simulink model "eml_2nd_order_filter_vectorized"  (Simulink 7.3)
settings: Solver=FixedStepDiscrete  StartTime=0.0  StopTime=0  RelTol=1e-3
values from neighbouring files (symbols this model uses):
  den = [1.0                0.0                0.171600341796875]    [fi_datatype_override_demo.m]    (also in numbercircle.m = den(ones(size(bin,1),1),:))
  num = [0.29290771484375   0.585784912109375  0.292907714843750]    [fi_datatype_override_demo.m]    (also in numbercircle.m = [bin equiv num2str(x)])
settings Model: Creator=tbryan  LastModifiedBy=sbatabya  ExtModeAutoUpdateStatusClock=off
settings OptimizationCC: IndividualOutputsThreshold=0  InitFltsAndDblsToZero=on
settings DebuggingCC: ArtificialAlgebraicLoopMsg=none  SignalResolutionControl=TryResolveAllWithWarning  SolverPrmCheckMsg=none  InheritedTsInSrcMsg=none  DiscreteInheritContinuousMsg=none  MultiTaskDSMMsg=warning  MultiTaskCondExecSysMsg=none  MultiTaskRateTransMsg=warning  TasksWithSamePriorityMsg=none  SigSpecEnsureSampleTimeMsg=none  IntegerOverflowMsg=none  Int32ToFloatConvMsg=none  ParameterDowncastMsg=none  ParameterOverflowMsg=none  ParameterPrecisionLossMsg=none  UnknownTsInhSupMsg=none
settings SFSimCC: SFSimOverflowDetection=off
settings RTWCC: GenerateReport=on  LaunchReport=on  IncludeERTFirstTime=on

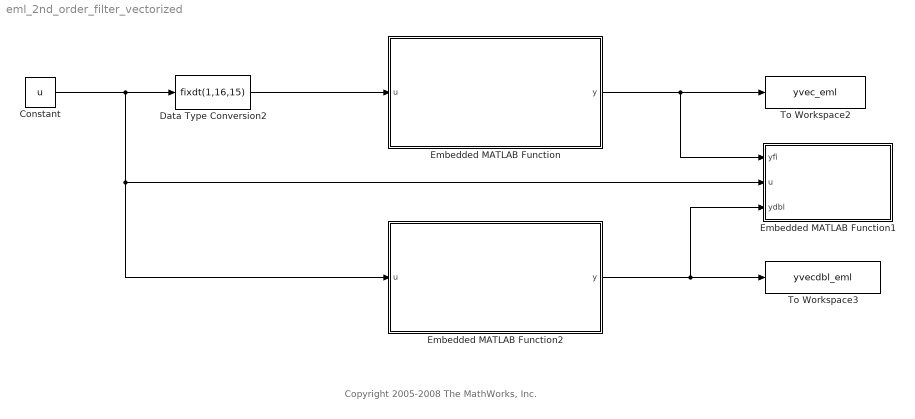
== system eml_2nd_order_filter_vectorized ==
  note: Copyright 2005-2008 The MathWorks, Inc.
  Constant : Constant  Value=u  OutDataTypeMode=double  OutDataType=sfix(16)  OutScaling=2^0  OutDataTypeStr=double
  Data Type Conversion2 : DataTypeConversion  OutDataTypeMode=Specify via dialog  OutDataType=fixdt(1,16,15)  OutDataTypeStr=fixdt(1,16,15)  RndMeth=Nearest  SaturateOnIntegerOverflow=on
  Embedded MATLAB Function : Stateflow chart
  Embedded MATLAB Function1 : Stateflow chart
  Embedded MATLAB Function2 : Stateflow chart
  To Workspace2 : ToWorkspace  VariableName=yvec_eml  SampleTime=-1  SaveFormat=Array
      settings: MaxDataPoints=1
  To Workspace3 : ToWorkspace  VariableName=yvecdbl_eml  SampleTime=-1  SaveFormat=Array
      settings: MaxDataPoints=1
  wires:
  Constant/1 -> Data Type Conversion2/1, Embedded MATLAB Function1/2(u), Embedded MATLAB Function2/1(u)
  Data Type Conversion2/1 -> Embedded MATLAB Function/1(u)
  Embedded MATLAB Function/1(y) -> To Workspace2/1, Embedded MATLAB Function1/1(yfi)
  Embedded MATLAB Function2/1(y) -> To Workspace3/1, Embedded MATLAB Function1/3(ydbl)

== matlab function Embedded MATLAB Function1 ==
  data: yfi input double; u input double; ydbl input double; num parameter double; den parameter double
function vector_plot(yfi, u, ydbl, num, den)

eml.extrinsic('fi_datatype_override_demo_plot');

fi_datatype_override_demo_plot(num,den,u,yfi,ydbl,'Embedded MATLAB Case')

== matlab function Embedded MATLAB Function2 ==
  data: num parameter double; den parameter double; u input double; y output double
function y = fi_2nd_order_filter(num, den, u)
%   Copyright 2005 The MathWorks, Inc.
%   $Revision: 1.1.6.4 $  $Date: 2008/12/01 07:13:09 $

y = fieml_2nd_order_filter(num,den,u);

== matlab function Embedded MATLAB Function ==
  data: num parameter double; den parameter double; u input double; y output double
function y = fi_2nd_order_filter(num, den, u)
%   Copyright 2005 The MathWorks, Inc.
%   $Revision: 1.1.6.4 $  $Date: 2008/12/01 07:13:09 $

y = fieml_2nd_order_filter(num,den,u);
